simulink model "nonlineardtm"  (R2018b)
settings: configuration reference "Physics" (kept outside this file)
model workspace (MAT data in the model file):
  MCOS : class17 (value not decoded)
undefined symbols (not defined in the file): INIT__initialvalues__Vehicle_InitialPitchAngle, INIT__initialvalues__Vehicle_InitialPitchRate_radps, INIT__initialvalues__Vehicle_InitialVelocity_mps__2, INIT__initialvalues__Vehicle_InitialVelocity_mps__3, INIT__initialvalues__Vehicle_InitialYawAngle, INIT__initialvalues__Vehicle_InitialYawRate_radps, tireFL__INERTIAL__m_Wheel_kg, tireFL__SCALING__LCX, tireFL__SCALING__LCY, tireFL__SCALING__LCZ, tireFL__SCALING__LEX, tireFL__SCALING__LEY, tireFL__SCALING__LFZO, tireFL__SCALING__LGAY, tireFL__SCALING__LGAZ, tireFL__SCALING__LHX, tireFL__SCALING__LHY, tireFL__SCALING__LKX, tireFL__SCALING__LKY, tireFL__SCALING__LMPHI, tireFL__SCALING__LMUV, tireFL__SCALING__LMX, tireFL__SCALING__LMY, tireFL__SCALING__LRES, tireFL__SCALING__LS, tireFL__SCALING__LTR, tireFL__SCALING__LVMX, tireFL__SCALING__LVX, tireFL__SCALING__LVY, tireFL__SCALING__LVYKA, tireFL__SCALING__LXAL, tireFL__SCALING__LYKA, tireFR__INERTIAL__m_Wheel_kg, tireFR__SCALING__LCX, tireFR__SCALING__LCY, tireFR__SCALING__LCZ, tireFR__SCALING__LEX, tireFR__SCALING__LEY, tireFR__SCALING__LFZO, tireFR__SCALING__LGAY, tireFR__SCALING__LGAZ, tireFR__SCALING__LHX, tireFR__SCALING__LHY, tireFR__SCALING__LKX, tireFR__SCALING__LKY, tireFR__SCALING__LMPHI, tireFR__SCALING__LMUV, tireFR__SCALING__LMX, tireFR__SCALING__LMY, tireFR__SCALING__LRES, tireFR__SCALING__LS, tireFR__SCALING__LTR, tireFR__SCALING__LVMX, tireFR__SCALING__LVX, tireFR__SCALING__LVY, tireFR__SCALING__LVYKA, tireFR__SCALING__LXAL, tireFR__SCALING__LYKA, tireRL__INERTIAL__m_Wheel_kg, tireRL__SCALING__LCX ... (+71)
libraries: vehdynlibtire_TUM x4, vehdynlibsuspension x2, vrlib x1, vehdynlibeom_TUM x1
(part 2 of 5)

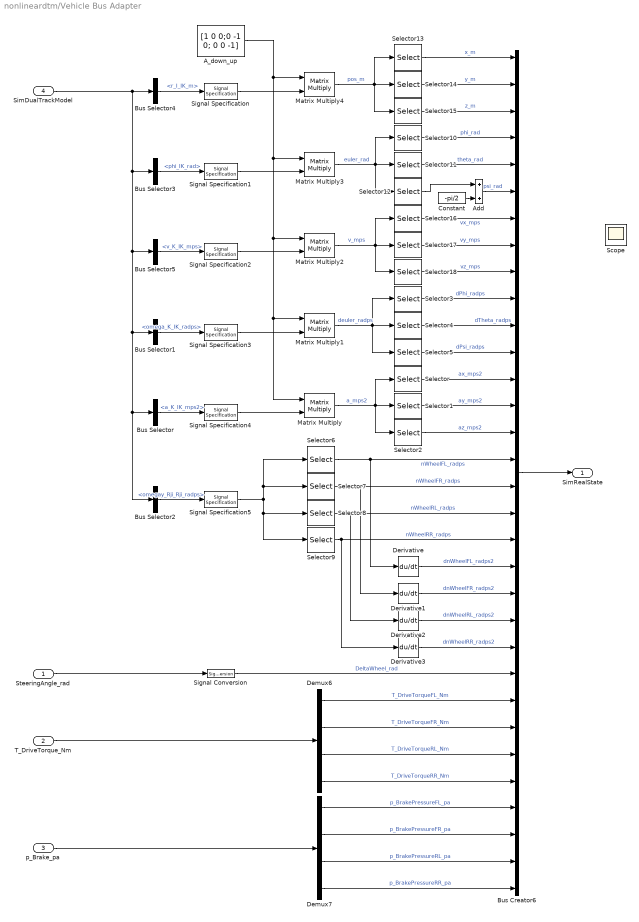
== system nonlineardtm/Vehicle Bus Adapter ==
  SteeringAngle_rad : Inport
  T_DriveTorque_Nm : Inport  Port=2
  "p_Brake_pa " : Inport  Port=3
  SimDualTrackModel : Inport  Port=4
  A_down_up : Constant  Value=[1 0 0;0 -1 0; 0 0 -1]
  Add : Sum
  Bus Creator6 : BusCreator  Inputs=32
  Bus Selector : BusSelector  OutputSignals=signal1.a_K_IK_mps2
  Bus Selector1 : BusSelector  OutputSignals=signal1.omega_K_IK_radps
  Bus Selector2 : BusSelector  OutputSignals=SimWheel.omegay_Rji_Rji_radps
  Bus Selector3 : BusSelector  OutputSignals=signal1.phi_IK_rad
  Bus Selector4 : BusSelector  OutputSignals=signal1.r_I_IK_m
  Bus Selector5 : BusSelector  OutputSignals=signal1.v_K_IK_mps
  Constant : Constant  Value=-pi/2
  Demux6 : Demux
  Demux7 : Demux
  Derivative{,1..3} (4 alike) : Derivative
  Matrix Multiply{,1..4} (5 alike) : Product  Multiplication=Matrix(*)
  Scope : Scope
  Selector{,3,10,13,16} (5 alike) : Selector  InputPortWidth=3  IndexOptions=Index vector (dialog)  Indices=[1]  OutputSizes=1
  Selector{1,4,11,14,17} (5 alike) : Selector  InputPortWidth=3  IndexOptions=Index vector (dialog)  Indices=[2]  OutputSizes=1
  Selector{2,5,12,15,18} (5 alike) : Selector  InputPortWidth=3  IndexOptions=Index vector (dialog)  Indices=[3]  OutputSizes=1
  Selector6 : Selector  InputPortWidth=4  IndexOptions=Index vector (dialog)  Indices=[1]  OutputSizes=1
  Selector7 : Selector  InputPortWidth=4  IndexOptions=Index vector (dialog)  Indices=[2]  OutputSizes=1
  Selector8 : Selector  InputPortWidth=4  IndexOptions=Index vector (dialog)  Indices=[3]  OutputSizes=1
  Selector9 : Selector  InputPortWidth=4  IndexOptions=Index vector (dialog)  Indices=4  OutputSizes=1
  Signal Conversion : SignalConversion  OverrideOpt=off
  Signal Specification{,1..4} (5 alike) : SignalSpecification  Dimensions=[3,1]
  Signal Specification5 : SignalSpecification  Dimensions=[1,4]
  SimRealState : Outport
  wires:
  Bus Selector4/1 -> Signal Specification/1  "<r_I_IK_m>"
  Matrix Multiply2/1 -> Selector18/1, Selector16/1, Selector17/1  "v_mps"
  Selector14/1 -> Bus Creator6/2  "y_m"
  Matrix Multiply/1 -> Selector2/1, Selector/1, Selector1/1  "a_mps2"
  Selector1/1 -> Bus Creator6/14  "ay_mps2"
  Bus Selector2/1 -> Signal Specification5/1  "<omegay_Rji_Rji_radps>"
  Selector16/1 -> Bus Creator6/7  "vx_mps"
  Selector17/1 -> Bus Creator6/8  "vy_mps"
  Selector9/1 -> Derivative3/1, Bus Creator6/19  "nWheelRR_radps"
  Bus Selector3/1 -> Signal Specification1/1  "<phi_IK_rad>"
  Add/1 -> Bus Creator6/6  "psi_rad"
  Bus Selector5/1 -> Signal Specification2/1  "<v_K_IK_mps>"
  Matrix Multiply1/1 -> Selector5/1, Selector3/1, Selector4/1  "deuler_radps"
  Selector6/1 -> Derivative/1, Bus Creator6/16  "nWheelFL_radps"
  SimDualTrackModel/1 -> Bus Selector2/1, Bus Selector/1, Bus Selector1/1, Bus Selector5/1, Bus Selector3/1, Bus Selector4/1
  Bus Selector1/1 -> Signal Specification3/1  "<omega_K_IK_radps>"
  Matrix Multiply4/1 -> Selector15/1, Selector13/1, Selector14/1  "pos_m"
  Matrix Multiply3/1 -> Selector12/1, Selector10/1, Selector11/1  "euler_rad"
  Selector7/1 -> Derivative1/1, Bus Creator6/17  "nWheelFR_radps"
  A_down_up/1 -> Matrix Multiply4/1, Matrix Multiply/1, Matrix Multiply1/1, Matrix Multiply2/1, Matrix Multiply3/1
  Selector10/1 -> Bus Creator6/4  "phi_rad"
  Selector15/1 -> Bus Creator6/3  "z_m"
  Selector8/1 -> Derivative2/1, Bus Creator6/18  "nWheelRL_radps"
  Bus Selector/1 -> Signal Specification4/1  "<a_K_IK_mps2>"
  Selector13/1 -> Bus Creator6/1  "x_m"
  Selector5/1 -> Bus Creator6/12  "dPsi_radps"
  Selector/1 -> Bus Creator6/13  "ax_mps2"
  Signal Specification/1 -> Matrix Multiply4/2
  Signal Specification1/1 -> Matrix Multiply3/2
  Signal Specification2/1 -> Matrix Multiply2/2
  Signal Specification3/1 -> Matrix Multiply1/2
  Signal Specification4/1 -> Matrix Multiply/2
  Signal Specification5/1 -> Selector9/1, Selector8/1, Selector7/1, Selector6/1
  Selector11/1 -> Bus Creator6/5  "theta_rad"
  Selector18/1 -> Bus Creator6/9  "vz_mps"
  Selector3/1 -> Bus Creator6/10  "dPhi_radps"
  Selector4/1 -> Bus Creator6/11  "dTheta_radps"
  Selector2/1 -> Bus Creator6/15  "az_mps2"
  Bus Creator6/1 -> SimRealState/1
  Constant/1 -> Add/2
  Selector12/1 -> Add/1
  SteeringAngle_rad/1 -> Signal Conversion/1
  Signal Conversion/1 -> Bus Creator6/24  "DeltaWheel_rad"
  Derivative/1 -> Bus Creator6/20  "dnWheelFL_radps2"
  Derivative1/1 -> Bus Creator6/21  "dnWheelFR_radps2"
  Derivative2/1 -> Bus Creator6/22  "dnWheelRL_radps2"
  Derivative3/1 -> Bus Creator6/23  "dnWheelRR_radps2"
  Demux7/4 -> Bus Creator6/32  "p_BrakePressureRR_pa"
  Demux7/1 -> Bus Creator6/29  "p_BrakePressureFL_pa"
  Demux6/1 -> Bus Creator6/25  "T_DriveTorqueFL_Nm"
  Demux7/3 -> Bus Creator6/31  "p_BrakePressureRL_pa"
  Demux6/3 -> Bus Creator6/27  "T_DriveTorqueRL_Nm"
  Demux6/2 -> Bus Creator6/26  "T_DriveTorqueFR_Nm"
  Demux7/2 -> Bus Creator6/30  "p_BrakePressureFR_pa"
  Demux6/4 -> Bus Creator6/28  "T_DriveTorqueRR_Nm"
  "p_Brake_pa "/1 -> Demux7/1
  T_DriveTorque_Nm/1 -> Demux6/1
